simulink model "FSM_parking_gate"  (R2024a)
settings: Solver=FixedStepAuto  StartTime=0.0  StopTime=100  FixedStep=0.2  RelTol=1e-3
settings Model: PacingRate=9  Creator=ArriGE66  LastModifiedBy=Bocchio
settings ModelReferenceCC: EnableRefExpFcnMdlSchedulingChecks=on
settings RTWCC: GPUComputeCapability=3.5

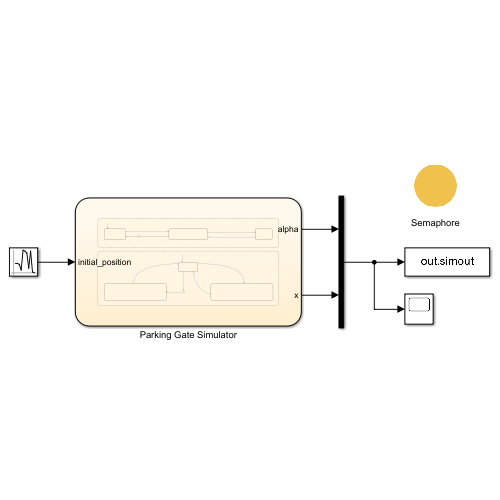
[thumbnail: Simulink's stored preview of the top-level diagram]
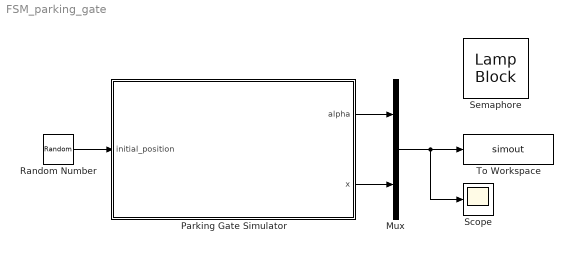
== system FSM_parking_gate ==
  Mux : Mux  Inputs=2
  Parking Gate Simulator : Stateflow chart  TreatAsAtomicUnit=on
  Random Number : RandomNumber  Mean=-15  Variance=5  SampleTime=0.2
  Scope : Scope
  Semaphore : LampBlock  LabelPosition=Hide  Icon=Circle
  To Workspace : ToWorkspace  VariableName=simout  SampleTime=-1
  wires:
  Random Number/1 -> Parking Gate Simulator/1(initial_position)
  Parking Gate Simulator/1(alpha) -> Mux/1
  Parking Gate Simulator/2(x) -> Mux/2
  Mux/1 -> To Workspace/1, Scope/1

== stateflow chart FSM_parking_gate/Parking Gate Simulator ==
  state Car [parallel]
    settings: executionOrder=1
    state Spawning
      entry:
      x = initial_position;
    state Moving
      during:
      v = min(abs(x), 30/3.6)  + 1e-1;
      x = min(x + v*dt, stop_x);
    state Waiting
      entry:
      v = 0;
    (default) -> Spawning
    Spawning -> Moving : {stop_x = gate_x}
    Moving -> Waiting [order 2] : [x == stop_x && ~gate_up]
    (junction 130) -> Spawning : after(2, sec)
    Moving -> (junction 130) [order 1] : [x > gate_x && ~gate_up]
    Waiting -> Moving : [gate_up]{stop_x = +inf}
  state Gate [parallel]
    settings: executionOrder=2
    state Idle
      entry:
      omega = 0;
    state Lowering
      during:
      omega = max(omega - max_omega_dot * dt, -max_omega);
      alpha = max(alpha + omega * dt, 0);
      exit:
      gate_up = false
    state Raising
      during:
      omega = min(omega + max_omega_dot * dt, max_omega);
      alpha = min(alpha + omega * dt, 90);
      exit:
      gate_up = true;
    (default) -> Idle : {gate_up = false}
    Lowering -> Idle : [alpha == 0]
    Idle -> Raising [order 2] : [in(Car.Waiting)]
    Idle -> (junction 120) [order 1] : [x > (gate_x + car_length) && gate_up]
    Raising -> Idle : [alpha == 90]
    (junction 120) -> Lowering : after(2, sec)
  state Name [parallel]
    settings: executionOrder=3
  data: initial_position input; omega local double =0; dt constant double =0.2; max_omega_dot constant double =1; max_omega constant double =4; v local; car_length constant double =3; data local; data1 local; data2 local; alpha output double =0; x output; stop_x local; gate_x constant double =0; gate_up local boolean
  events: event local FUNCTION_CALL_EVENT; event1 local FUNCTION_CALL_EVENT; event2 local FUNCTION_CALL_EVENT; event3 local FUNCTION_CALL_EVENT
